simulink model "DWT"  (R2020a)
settings: Solver=ode45  StartTime=0.0  StopTime=4096+1024+100  RelTol=1e-3  EnableMultiTasking=on
PreLoadFcn:
  | xlrequire('imageData.mat'); xlrequire('PreLoadFcn');
PostLoadFcn:
  | open_system('DWT/Processor/Memory Controller','force'); pause(0.50); open_system('DWT');pause(0.50); close_system('DWT/Processor/Memory Controller');pause(0.50); close_system('DWT/Processor');
StopFcn:
  | xlrequire('StopFcn');
undefined symbols (not defined in the file or in its folder): b1Init, b2Init
libraries: xbsIndex_r4 x213, dspindex x4, dspsnks4 x2, dspmtrx3 x2, xbsCopyrightNotice_r4 x1, dspsrcs4 x1
(part 1 of 2)
settings Model: Creator=alexc  LastModifiedBy=viswanad
settings DataIOCC: LimitDataPoints=on  SaveFormat=Array  SignalLoggingSaveFormat=ModelDataLogs  ReturnWorkspaceOutputs=off  SignalLoggingName=sigsOut
settings OptimizationCC: BlockReduction=off  BooleanDataType=off  DefaultParameterBehavior=Inlined  ExpressionDepthLimit=2147483647  InitFltsAndDblsToZero=on  LifeSpan=inf
settings DebuggingCC: SaveWithParameterizedLinksMsg=none  UnderspecifiedInitializationDetection=Classic  MergeDetectMultiDrivingBlocksExec=none  SignalResolutionControl=TryResolveAllWithWarning  MultiTaskDSMMsg=warning  MultiTaskCondExecSysMsg=none  FcnCallInpInsideContextMsg=warning  AllowSymbolicDim=off  StateNameClashWarn=warning  SFUnexpectedBacktrackingDiag=warning  SFNoUnconditionalDefaultTransitionDiag=warning  SFExecutionAtInitializationDiag=none  ArithmeticOperatorsInVariantConditions=warning
settings HardwareCC: ProdBitPerPointer=32  ProdBitPerSizeT=32  ProdBitPerPtrDiffT=32  ProdLargestAtomicFloat=None  ProdIntDivRoundTo=Undefined  ProdEndianess=Unspecified  ProdWordSize=32  ProdHWDeviceType=32-bit Generic  TargetUnknown=on
settings ModelReferenceCC: PropagateSignalLabelsOutOfModel=off
settings SFSimCC: SimUseLocalCustomCode=off  CustomCodeUndefinedFunction=UseInterfaceOnly
settings RTWCC: Description=Generic Real-Time Target  RTWUseLocalCustomCode=off
settings CodeAppCC: StateflowObjectComments=on
settings GRTTargetCC: TargetFcnLib=ansi_tfl_tmw.mat  TargetLangStandard=C89/C90 (ANSI)  CombineOutputUpdateFcns=off  GRTInterface=on
settings ConfigComp: CovMetricSettings=dw  CovSaveCumulativeToWorkspaceVar=on  CovSaveSingleToWorkspaceVar=on  CovExternalEMLEnable=off

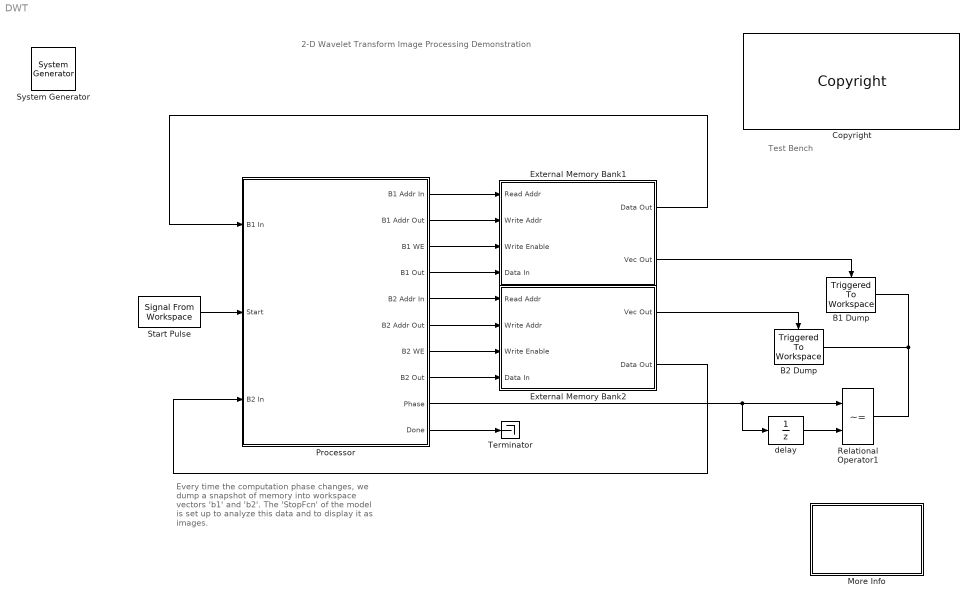
== system DWT ==
  note: Test
      |  Bench
  note: Every time the computation phase
      | changes, we dump a snapshot of
      | memory into workspace vectors  'b1'
      | and  'b2'.
      |
      | The 'StopFcn' of the model is set up
      | to analyze this data and to display
      | it as images.
  note: 2-D Wavelet Transform
      |  Image Processing Demonstration
  " System Generator" : xbsIndex_r4/ System Generator  Tag=genX  xilinxfamily=Kintex7  part=xc7k325t  speed=-3  package=fbg676  synthesis_tool=Vivado  clock_wrapper=Clock Enables  directory=./netlist  proj_type=Vivado  Synth_file=Vivado Synthesis Defaults  Impl_file=Vivado Implementation Defaults  testbench=off  simulink_period=1  sysclk_period=6  dcm_input_clock_period=10  incr_netlist=off  trim_vbits=Everywhere in SubSystem  dbl_ovrd=According to Block Masks  core_generation=According to Block Masks  run_coregen=off  deprecated_control=off  eval_field=0  block_type=sysgen
  B1 Dump : dspsnks4/Triggered To Workspace  TriggerType=Falling edge  VariableName=b1  Buffer=1000  Save2DMode=3-D array (concatenate along third dimension)
      settings: SourceProductBaseCode=DS  FixptAsFi=off
  B2 Dump : dspsnks4/Triggered To Workspace  TriggerType=Falling edge  VariableName=b2  Buffer=1000  Save2DMode=3-D array (concatenate along third dimension)
      settings: SourceProductBaseCode=DS  FixptAsFi=off
  Copyright : xbsCopyrightNotice_r4/Copyright  copyrighttext="Copyright (c) 2021  by  Xilinx, Inc. All rights reserved.<br><br>This file contains proprietary, confidential information of Xilinx, Inc., is distributed under license from Xilinx, Inc., and may be used, copied and/or disclosed only pursuant to the terms of a valid license agreement with Xilinx, Inc. Xilinx hereby grants you a license to use this file solely for design, simulation, implementation and creation of design files limited to Xilinx devices or technologies. Use with non-Xilinx devices or technologies is expressly prohibited and immediately terminates your license unless covered by a separate agreement.<br><br>Xilinx is providing this design, code, or information \"as-is\" solely for use in developing programs and solutions for Xilinx devices, with no obligation on the part of Xilinx to provide support. By providing this design, code, or information as one possible implementation of this feature, application or standard, Xilinx is making no representation that this implementation is free from any claims of infringement. You are responsible for obtaining any rights you may require for your implementation. Xilinx expressly disclaims any warranty whatsoever with respect to the adequacy of the implementation, including but not limited to any warranties or representations that this implementation is free from claims of infringement, implied warranties of merchantability or fitness for a particular purpose.<br><br>Xilinx products are not intended for use in life support appliances, devices, or systems. Use in such applications is expressly prohibited.<br><br>Any modifications that are made to the Source Code are done at the user's sole risk and will be unsupported.<br><br>This copyright and support notice must be retained as part of this text at all times. (c) Copyright 1995-2021 Xilinx, Inc. All rights reserved."  block_type=copyright
  External Memory Bank1 : Subsystem  mask{depth=size (b2Init, 2), init_vec=b1Init}
      mask prompts: depth "Memory Depth"; init_vec "Initial Value"
  External Memory Bank2 : Subsystem  mask{depth=size (b2Init, 2), init_vec=b2Init}
      mask prompts: depth "Memory Depth"; init_vec "Initial Value"
  More Info : Subsystem
      mask Display: disp('Double click\n for\n more information.')
  Processor : Subsystem
  Relational Operator1 : RelationalOperator  Operator=~=  RndMeth=Nearest  InputSameDT=on
  Start Pulse : dspsrcs4/Signal From Workspace  X=[ 0 0 0 1 0 0]  Ts=1  nsamps=1  OutputAfterFinalValue=Setting to zero  ignoreOrWarnInputAndFrameLengths=off  OutputFrames=on
  Terminator : Terminator
  delay : UnitDelay  InitialCondition=-1  HasFrameUpgradeWarning=on
  wires:
  Processor/4(B1 Out) -> External Memory Bank1/4(Data In)
  Processor/3(B1 WE) -> External Memory Bank1/3(Write Enable)
  Processor/2(B1 Addr Out) -> External Memory Bank1/2(Write Addr)
  Processor/1(B1 Addr In) -> External Memory Bank1/1(Read Addr)
  Processor/5(B2 Addr In) -> External Memory Bank2/1(Read Addr)
  Processor/6(B2 Addr Out) -> External Memory Bank2/2(Write Addr)
  Processor/7(B2 WE) -> External Memory Bank2/3(Write Enable)
  Processor/8(B2 Out) -> External Memory Bank2/4(Data In)
  External Memory Bank1/1(Data Out) -> Processor/1(B1 In)
  External Memory Bank2/2(Data Out) -> Processor/3(B2 In)
  External Memory Bank2/1(Vec Out) -> B2 Dump/1
  External Memory Bank1/2(Vec Out) -> B1 Dump/1
  Processor/9(Phase) -> Relational Operator1/1, delay/1
  delay/1 -> Relational Operator1/2
  Relational Operator1/1 -> B1 Dump/Trigger, B2 Dump/Trigger
  Start Pulse/1 -> Processor/2(Start)
  Processor/10(Done) -> Terminator/1

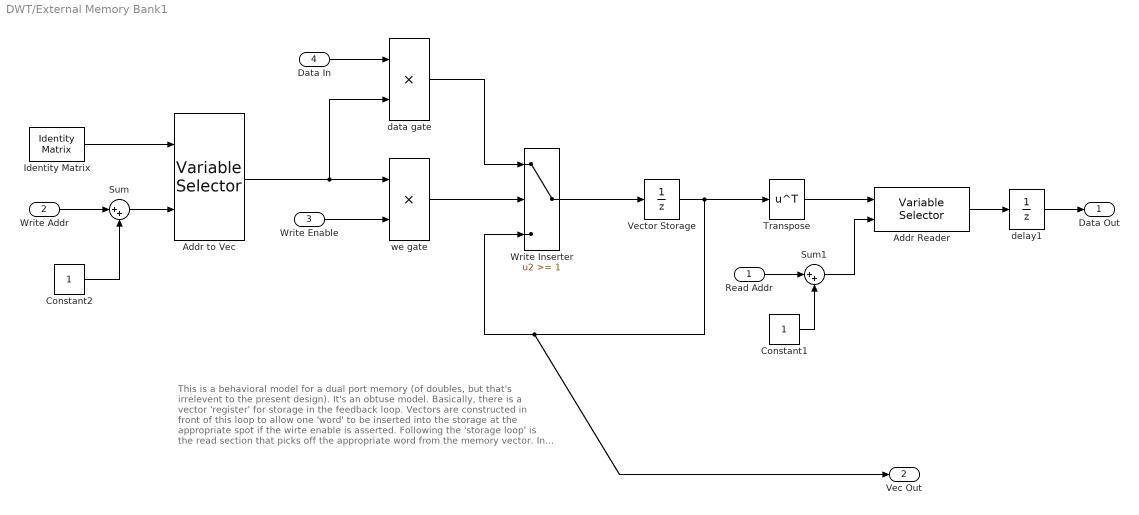
== system DWT/External Memory Bank1 ==
  note: This is a behavioral model for a dual port memory
      | (of doubles, but that's irrelevent to the present design).
      | It's an obtuse model.  Basically, there is a vector 'register'
      | for storage in the feedback loop. Vectors are constructed
      | in front of this loop to allow one 'word' to be inserted into the
      | storage  at the appropriate spot if the wirte enable is
      | asserted.  Following the 'storage loop' is the read section
      | that picks off the appropriate word from the memory vector.
      |
      | In case of overlapping addresss, the read is done before
      | the write changes the stored word.
      |
      | At every time step, the full contents of the memory are output
      | as a  vector of doubles.  This is a very handy  feature  for
      | analysis and debugging.
  Read Addr : Inport
  Write Addr : Inport  Port=2
  Write Enable : Inport  Port=3
  Data In : Inport  Port=4
  Addr Reader : dspindex/Variable Selector  NumInputs=1  rowsOrCols=Rows  IdxMode=Variable  Elements=[1 3]  ZerOneIdxMode=One-based  errmode=Generate Error  FillMode=on  FillValues=0
  Addr to Vec : dspindex/Variable Selector  NumInputs=1  rowsOrCols=Rows  IdxMode=Variable  Elements=[1 3]  ZerOneIdxMode=One-based  errmode=Clip Index  FillMode=on  FillValues=0
  Constant1 : Constant
  Constant2 : Constant
  Identity Matrix : dspmtrx3/Identity Matrix  Inherit=off  N=depth  Ts=1  dataType=double  isSigned=on  wordLen=16  udDataType=sfix(16)  fracBitsMode=Best precision  numFracBits=15  OutDataTypeStr=double  LastOutDataTypeStr=double
  Sum : Sum  Inputs=|++  InputSameDT=on  SaturateOnIntegerOverflow=on  OutDataTypeStr=Inherit: Same as first input
  Sum1 : Sum  Inputs=|++  InputSameDT=on  SaturateOnIntegerOverflow=on  OutDataTypeStr=Inherit: Same as first input
  Transpose : Math  Operator=transpose  SaturateOnIntegerOverflow=on
  Vector Storage : UnitDelay  InitialCondition=init_vec  HasFrameUpgradeWarning=on
  Write Inserter : Switch  Threshold=1  SaturateOnIntegerOverflow=on  InputSameDT=on
  data gate : Product  InputSameDT=on  SaturateOnIntegerOverflow=on  OutDataTypeStr=Inherit: Same as first input
  delay1 : UnitDelay  HasFrameUpgradeWarning=on
  we gate : Product  InputSameDT=on  SaturateOnIntegerOverflow=on  OutDataTypeStr=Inherit: Same as first input
  Data Out : Outport  VectorParamsAs1DForOutWhenUnconnected=off
  Vec Out : Outport  Port=2  VectorParamsAs1DForOutWhenUnconnected=off
  wires:
  Write Inserter/1 -> Vector Storage/1
  Addr Reader/1 -> delay1/1
  Addr to Vec/1 -> we gate/1, data gate/2
  Identity Matrix/1 -> Addr to Vec/1
  Write Enable/1 -> we gate/2
  Transpose/1 -> Addr Reader/1
  Data In/1 -> data gate/1
  we gate/1 -> Write Inserter/2
  data gate/1 -> Write Inserter/1
  Sum/1 -> Addr to Vec/2
  Write Addr/1 -> Sum/1
  Constant2/1 -> Sum/2
  Constant1/1 -> Sum1/2
  Sum1/1 -> Addr Reader/2
  delay1/1 -> Data Out/1
  Vector Storage/1 -> Transpose/1, Vec Out/1, Write Inserter/3
  Read Addr/1 -> Sum1/1

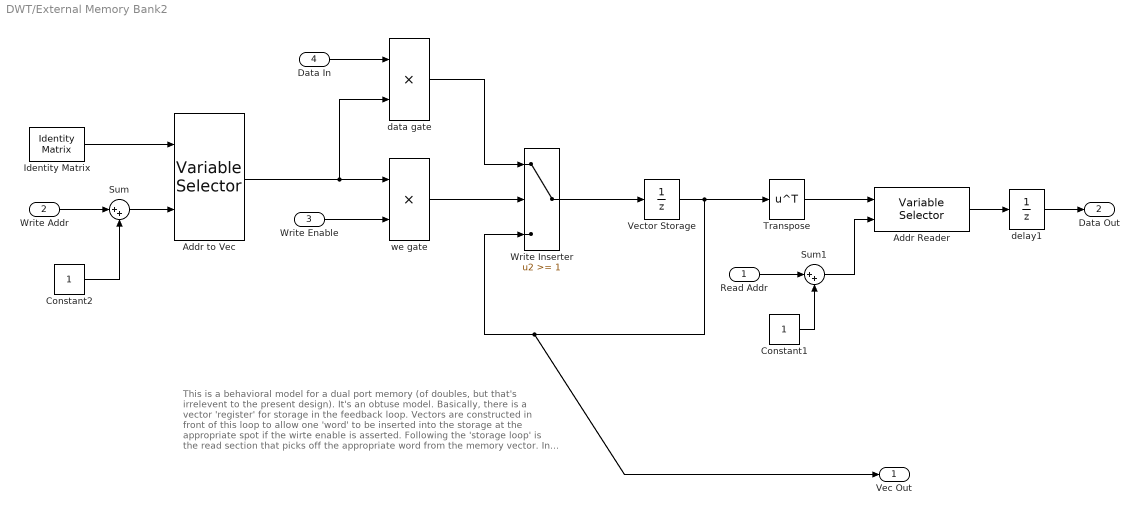
== system DWT/External Memory Bank2 ==
  note: This is a behavioral model for a dual port memory
      | (of doubles, but that's irrelevent to the present design).
      | It's an obtuse model.  Basically, there is a vector 'register'
      | for storage in the feedback loop. Vectors are constructed
      | in front of this loop to allow one 'word' to be inserted into the
      | storage  at the appropriate spot if the wirte enable is
      | asserted.  Following the 'storage loop' is the read section
      | that picks off the appropriate word from the memory vector.
      |
      | In case of overlapping addresss, the read is done before
      | the write changes the stored word.
      |
      | At every time step, the full contents of the memory are output
      | as a  vector of doubles.  This is a very handy  feature  for
      | analysis and debugging.
  Read Addr : Inport
  Write Addr : Inport  Port=2
  Write Enable : Inport  Port=3
  Data In : Inport  Port=4
  Addr Reader : dspindex/Variable Selector  NumInputs=1  rowsOrCols=Rows  IdxMode=Variable  Elements=[1 3]  ZerOneIdxMode=One-based  errmode=Clip Index  FillMode=on  FillValues=0
  Addr to Vec : dspindex/Variable Selector  NumInputs=1  rowsOrCols=Rows  IdxMode=Variable  Elements=[1 3]  ZerOneIdxMode=One-based  errmode=Clip Index  FillMode=on  FillValues=0
  Constant1 : Constant
  Constant2 : Constant
  Identity Matrix : dspmtrx3/Identity Matrix  Inherit=off  N=depth  Ts=1  dataType=double  isSigned=on  wordLen=16  udDataType=sfix(16)  fracBitsMode=Best precision  numFracBits=15  OutDataTypeStr=double  LastOutDataTypeStr=double
  Sum : Sum  Inputs=|++  InputSameDT=on  SaturateOnIntegerOverflow=on  OutDataTypeStr=Inherit: Same as first input
  Sum1 : Sum  Inputs=|++  InputSameDT=on  SaturateOnIntegerOverflow=on  OutDataTypeStr=Inherit: Same as first input
  Transpose : Math  Operator=transpose  SaturateOnIntegerOverflow=on
  Vector Storage : UnitDelay  InitialCondition=init_vec  HasFrameUpgradeWarning=on
  Write Inserter : Switch  Threshold=1  SaturateOnIntegerOverflow=on  InputSameDT=on
  data gate : Product  InputSameDT=on  SaturateOnIntegerOverflow=on  OutDataTypeStr=Inherit: Same as first input
  delay1 : UnitDelay  HasFrameUpgradeWarning=on
  we gate : Product  InputSameDT=on  SaturateOnIntegerOverflow=on  OutDataTypeStr=Inherit: Same as first input
  Vec Out : Outport  VectorParamsAs1DForOutWhenUnconnected=off
  Data Out : Outport  Port=2  VectorParamsAs1DForOutWhenUnconnected=off
  wires:
  Vector Storage/1 -> Transpose/1, Vec Out/1, Write Inserter/3
  delay1/1 -> Data Out/1
  Sum1/1 -> Addr Reader/2
  Read Addr/1 -> Sum1/1
  Constant1/1 -> Sum1/2
  Constant2/1 -> Sum/2
  Write Addr/1 -> Sum/1
  Sum/1 -> Addr to Vec/2
  data gate/1 -> Write Inserter/1
  we gate/1 -> Write Inserter/2
  Data In/1 -> data gate/1
  Transpose/1 -> Addr Reader/1
  Write Enable/1 -> we gate/2
  Identity Matrix/1 -> Addr to Vec/1
  Addr to Vec/1 -> data gate/2, we gate/1
  Addr Reader/1 -> delay1/1
  Write Inserter/1 -> Vector Storage/1

== system DWT/More Info ==
  note: The test bench for this wavelet design consists of a processor and behavioral models for a pair of external, dual-port memories.
      | The two memories are initialized with the pixel values of a grey-scale image.
      | The pixels from the initial image are interleaved into the two banks in a column first indexing strategy.
      | If the image contained a checkerboard of black and white pixels, then all of the black pixels will end up in the one bank, and all of
      | the white pixels in the other.  The processor includes a memory controller that schedules the reads and writes to memory, and
      | an image processing filter kernel that computes the 2D DWT decomposition of the image.  The processor has been configured
      | to compute two levels of decomposition on a 64 x 64 pixel image. The computation is done "in place" in the single image memory
      | space, and the initial pixel ordering is preserved throughout.
      |
      | A full color version of the design would easily fit in the same part as only the DWT datapath would require replication (the memoy
      | control could remain unchanged).
  note: 2-D Wavelet Transform Image Processing Demonstration

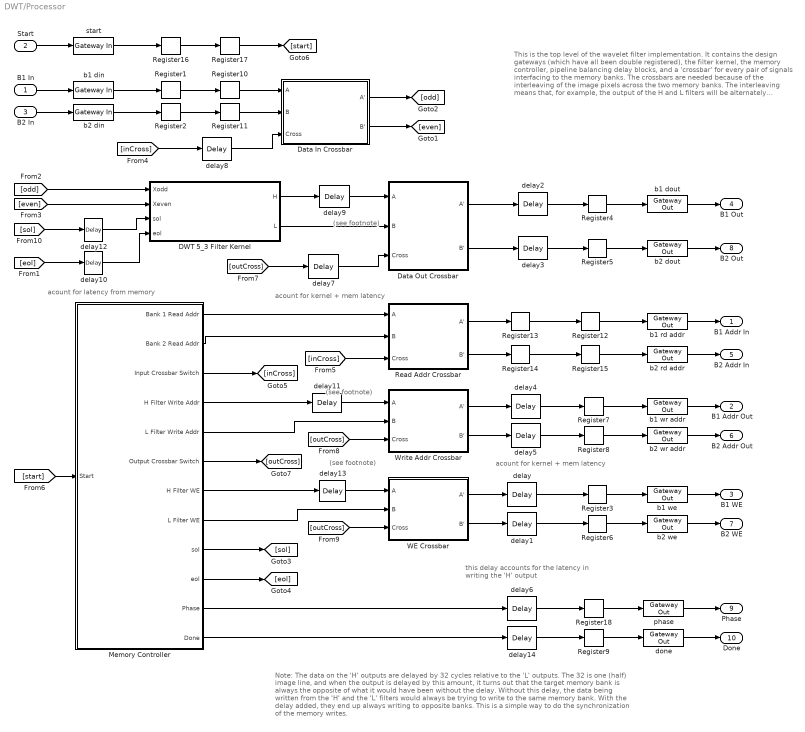
== system DWT/Processor ==
  note: This is the top level of the wavelet filter implementation.
      | It contains the design gateways (which have all been double
      | registered),  the filter kernel, the memory controller, pipeline
      | balancing delay blocks, and a 'crossbar' for every pair of signals
      | interfacing to the memory banks.  The crossbars are needed
      | because of the interleaving of the image pixels across the two
      | memory banks.  The interleaving means that, for example,
      | the output of the H and L filters will be alternately distributed
      | to the two memory banks.
  note: (see footnote)
  note: (see footnote)
  note: (see footnote)
  note: Note: The data on the 'H' outputs are delayed by 32 cycles relative to the 'L' outputs.
      | The 32 is one (half) image line, and when the output is delayed by this amount, it
      | turns out that the target memory bank is always the opposite of what it would have
      | been without the delay.  Without this delay, the data being written from the 'H' and
      | the 'L' filters would always be trying to write to the same memory bank.  With the
      | delay added, they end up always writing to opposite banks.  This is a simple way
      | to do the synchronization of the memory writes.
  note: this delay accounts for
      | the latency in writing the 'H' output
  note: acount for latency from memory
  note: acount for kernel + mem latency
  note: acount for kernel + mem latency
  B1 In : Inport
  Start : Inport  Port=2
  B2 In : Inport  Port=3
  DWT 5_3 Filter Kernel : Subsystem
  Data In Crossbar : Subsystem
  Data Out Crossbar : Subsystem
  Memory Controller : Subsystem  mask{N=6, M=6}
      mask prompts: N "Log Base 2 of Image Width"; M "Log Base 2 of Image Height"
  Read Addr Crossbar : Subsystem
  Register{1..18} (18 alike) : xbsIndex_r4/Register  init=0  rst=off  en=off  dbl_ovrd=off  block_type=register
  WE Crossbar : Subsystem
  Write Addr Crossbar : Subsystem
  b1 din : xbsIndex_r4/Gateway In  gui_display_data_type=Fixed-point  arith_type="Signed  (2's comp)"  n_bits=10  bin_pt=0  preci_type=Single  exp_width=8  frac_width=24  rows=1  columns=1  quantization="Round  (unbiased: +/- Inf)"  overflow=Saturate  period=1  UseAsADC=off  ADCChannel='1'  interface=None  automatic_assignment=on  address_offset=hex2dec('00')  intf_name=''  intf_description=''  default_value=0  timing_constraint=None  locs_specified=off  LOCs={}  io_standard={}  inherit_from_input=off  hdl_port=on  dbl_ovrd=off  block_type=gatewayin
  b1 dout : xbsIndex_r4/Gateway Out  inherit_from_input=off  hdl_port=on  rows=1  columns=1  UseAsDAC=off  DACChannel='1'  interface=None  automatic_assignment=on  address_offset=hex2dec('00')  intf_name=''  intf_description=''  timing_constraint=None  locs_specified=off  LOCs={}  io_standard={}  block_type=gatewayout
  b1 rd addr : xbsIndex_r4/Gateway Out  inherit_from_input=off  hdl_port=on  rows=1  columns=1  UseAsDAC=off  DACChannel='1'  interface=None  automatic_assignment=on  address_offset=hex2dec('00')  intf_name=''  intf_description=''  timing_constraint=None  locs_specified=off  LOCs={}  io_standard={}  block_type=gatewayout
  b1 we : xbsIndex_r4/Gateway Out  inherit_from_input=off  hdl_port=on  rows=1  columns=1  UseAsDAC=off  DACChannel='1'  interface=None  automatic_assignment=on  address_offset=hex2dec('00')  intf_name=''  intf_description=''  timing_constraint=None  locs_specified=off  LOCs={}  io_standard={}  block_type=gatewayout
  b1 wr addr : xbsIndex_r4/Gateway Out  inherit_from_input=off  hdl_port=on  rows=1  columns=1  UseAsDAC=off  DACChannel='1'  interface=None  automatic_assignment=on  address_offset=hex2dec('00')  intf_name=''  intf_description=''  timing_constraint=None  locs_specified=off  LOCs={}  io_standard={}  block_type=gatewayout
  b2 din : xbsIndex_r4/Gateway In  gui_display_data_type=Fixed-point  arith_type="Signed  (2's comp)"  n_bits=10  bin_pt=0  preci_type=Single  exp_width=8  frac_width=24  rows=1  columns=1  quantization="Round  (unbiased: +/- Inf)"  overflow=Saturate  period=1  UseAsADC=off  ADCChannel='1'  interface=None  automatic_assignment=on  address_offset=hex2dec('00')  intf_name=''  intf_description=''  default_value=0  timing_constraint=None  locs_specified=off  LOCs={}  io_standard={}  inherit_from_input=off  hdl_port=on  dbl_ovrd=off  block_type=gatewayin
  b2 dout : xbsIndex_r4/Gateway Out  inherit_from_input=off  hdl_port=on  rows=1  columns=1  UseAsDAC=off  DACChannel='1'  interface=None  automatic_assignment=on  address_offset=hex2dec('00')  intf_name=''  intf_description=''  timing_constraint=None  locs_specified=off  LOCs={}  io_standard={}  block_type=gatewayout
  b2 rd addr : xbsIndex_r4/Gateway Out  inherit_from_input=off  hdl_port=on  rows=1  columns=1  UseAsDAC=off  DACChannel='1'  interface=None  automatic_assignment=on  address_offset=hex2dec('00')  intf_name=''  intf_description=''  timing_constraint=None  locs_specified=off  LOCs={}  io_standard={}  block_type=gatewayout
  b2 we : xbsIndex_r4/Gateway Out  inherit_from_input=off  hdl_port=on  rows=1  columns=1  UseAsDAC=off  DACChannel='1'  interface=None  automatic_assignment=on  address_offset=hex2dec('00')  intf_name=''  intf_description=''  timing_constraint=None  locs_specified=off  LOCs={}  io_standard={}  block_type=gatewayout
  b2 wr addr : xbsIndex_r4/Gateway Out  inherit_from_input=off  hdl_port=on  rows=1  columns=1  UseAsDAC=off  DACChannel='1'  interface=None  automatic_assignment=on  address_offset=hex2dec('00')  intf_name=''  intf_description=''  timing_constraint=None  locs_specified=off  LOCs={}  io_standard={}  block_type=gatewayout
  delay{,1,4..5} (4 alike) : xbsIndex_r4/Delay  rst=off  infoeditControl=Selection of Reset will increase slice count due to use of real FFs and instead of SRLs  en=off  latency=15  reg_retiming=off  dbl_ovrd=off  block_type=delay
  delay10 : xbsIndex_r4/Delay  rst=off  infoeditControl=Selection of Reset will increase slice count due to use of real FFs and instead of SRLs  en=off  latency=6  reg_retiming=off  dbl_ovrd=off  block_type=delay
  delay11 : xbsIndex_r4/Delay  rst=off  infoeditControl=Selection of Reset will increase slice count due to use of real FFs and instead of SRLs  en=off  latency=32  reg_retiming=off  dbl_ovrd=off  block_type=delay
  delay12 : xbsIndex_r4/Delay  rst=off  infoeditControl=Selection of Reset will increase slice count due to use of real FFs and instead of SRLs  en=off  latency=6  reg_retiming=off  dbl_ovrd=off  block_type=delay
  delay13 : xbsIndex_r4/Delay  rst=off  infoeditControl=Selection of Reset will increase slice count due to use of real FFs and instead of SRLs  en=off  latency=32  reg_retiming=off  dbl_ovrd=off  block_type=delay
  delay14 : xbsIndex_r4/Delay  rst=off  infoeditControl=Selection of Reset will increase slice count due to use of real FFs and instead of SRLs  en=off  latency=32+15  reg_retiming=off  dbl_ovrd=off  block_type=delay
  delay2 : xbsIndex_r4/Delay  rst=off  infoeditControl=Selection of Reset will increase slice count due to use of real FFs and instead of SRLs  en=off  latency=1  reg_retiming=off  dbl_ovrd=off  block_type=delay
  delay3 : xbsIndex_r4/Delay  rst=off  infoeditControl=Selection of Reset will increase slice count due to use of real FFs and instead of SRLs  en=off  latency=1  reg_retiming=off  dbl_ovrd=off  block_type=delay
  delay6 : xbsIndex_r4/Delay  rst=off  infoeditControl=Selection of Reset will increase slice count due to use of real FFs and instead of SRLs  en=off  latency=32+15  reg_retiming=off  dbl_ovrd=off  block_type=delay
  delay7 : xbsIndex_r4/Delay  rst=off  infoeditControl=Selection of Reset will increase slice count due to use of real FFs and instead of SRLs  en=off  latency=14  reg_retiming=off  dbl_ovrd=off  block_type=delay
  delay8 : xbsIndex_r4/Delay  rst=off  infoeditControl=Selection of Reset will increase slice count due to use of real FFs and instead of SRLs  en=off  latency=6  reg_retiming=off  dbl_ovrd=off  block_type=delay
  delay9 : xbsIndex_r4/Delay  rst=off  infoeditControl=Selection of Reset will increase slice count due to use of real FFs and instead of SRLs  en=off  latency=32  reg_retiming=off  dbl_ovrd=off  block_type=delay
  done : xbsIndex_r4/Gateway Out  inherit_from_input=off  hdl_port=on  rows=1  columns=1  UseAsDAC=off  DACChannel='1'  interface=None  automatic_assignment=on  address_offset=hex2dec('00')  intf_name=''  intf_description=''  timing_constraint=None  locs_specified=off  LOCs={}  io_standard={}  block_type=gatewayout
  phase : xbsIndex_r4/Gateway Out  inherit_from_input=off  hdl_port=on  rows=1  columns=1  UseAsDAC=off  DACChannel='1'  interface=None  automatic_assignment=on  address_offset=hex2dec('00')  intf_name=''  intf_description=''  timing_constraint=None  locs_specified=off  LOCs={}  io_standard={}  block_type=gatewayout
  start : xbsIndex_r4/Gateway In  gui_display_data_type=Boolean  arith_type=Boolean  n_bits=1  bin_pt=0  preci_type=Single  exp_width=8  frac_width=24  rows=1  columns=1  quantization="Round  (unbiased: +/- Inf)"  overflow=Saturate  period=1  UseAsADC=off  ADCChannel='1'  interface=None  automatic_assignment=on  address_offset=hex2dec('00')  intf_name=''  intf_description=''  default_value=0  timing_constraint=None  locs_specified=off  LOCs={}  io_standard={}  inherit_from_input=off  hdl_port=on  dbl_ovrd=off  block_type=gatewayin
  B1 Addr In : Outport  VectorParamsAs1DForOutWhenUnconnected=off
  B1 Addr Out : Outport  Port=2  VectorParamsAs1DForOutWhenUnconnected=off
  B1 WE : Outport  Port=3  VectorParamsAs1DForOutWhenUnconnected=off
  B1 Out : Outport  Port=4  VectorParamsAs1DForOutWhenUnconnected=off
  B2 Addr In : Outport  Port=5  VectorParamsAs1DForOutWhenUnconnected=off
  B2 Addr Out : Outport  Port=6  VectorParamsAs1DForOutWhenUnconnected=off
  B2 WE : Outport  Port=7  VectorParamsAs1DForOutWhenUnconnected=off
  B2 Out : Outport  Port=8  VectorParamsAs1DForOutWhenUnconnected=off
  Phase : Outport  Port=9  VectorParamsAs1DForOutWhenUnconnected=off
  Done : Outport  Port=10  VectorParamsAs1DForOutWhenUnconnected=off
  wires:
  b1 din/1 -> Register1/1
  b2 din/1 -> Register2/1
  [sol] -> delay12/1
  [eol] -> delay10/1
  [odd] -> DWT 5_3 Filter Kernel/1(Xodd)
  [even] -> DWT 5_3 Filter Kernel/2(Xeven)
  Register1/1 -> Register10/1
  Register2/1 -> Register11/1
  Memory Controller/5(L Filter Write Addr) -> Write Addr Crossbar/2(B)
  Memory Controller/4(H Filter Write Addr) -> delay11/1
  Memory Controller/11(Phase) -> delay6/1
  Memory Controller/9(sol) -> [sol]
  Memory Controller/10(eol) -> [eol]
  Write Addr Crossbar/1(A') -> delay4/1
  Write Addr Crossbar/2(B') -> delay5/1
  DWT 5_3 Filter Kernel/1(H) -> delay9/1
  DWT 5_3 Filter Kernel/2(L) -> Data Out Crossbar/2(B)
  Data Out Crossbar/1(A') -> delay2/1
  Data Out Crossbar/2(B') -> delay3/1
  Register4/1 -> b1 dout/1
  Register5/1 -> b2 dout/1
  b2 rd addr/1 -> B2 Addr In/1
  b1 wr addr/1 -> B1 Addr Out/1
  b2 wr addr/1 -> B2 Addr Out/1
  B1 In/1 -> b1 din/1
  B2 In/1 -> b2 din/1
  b1 dout/1 -> B1 Out/1
  b2 dout/1 -> B2 Out/1
  b1 we/1 -> B1 WE/1
  b2 we/1 -> B2 WE/1
  delay2/1 -> Register4/1
  delay3/1 -> Register5/1
  delay5/1 -> Register8/1
  delay4/1 -> Register7/1
  Register7/1 -> b1 wr addr/1
  Register8/1 -> b2 wr addr/1
  phase/1 -> Phase/1
  Data In Crossbar/1(A') -> [odd]
  Data In Crossbar/2(B') -> [even]
  Memory Controller/3(Input Crossbar Switch) -> [inCross]
  Read Addr Crossbar/1(A') -> Register13/1
  Read Addr Crossbar/2(B') -> Register14/1
  Memory Controller/2(Bank 2 Read Addr) -> Read Addr Crossbar/2(B)
  Memory Controller/1(Bank 1 Read Addr) -> Read Addr Crossbar/1(A)
  delay6/1 -> Register18/1
  delay7/1 -> Data Out Crossbar/3(Cross)
  delay8/1 -> Data In Crossbar/3(Cross)
  [inCross] -> delay8/1
  [inCross] -> Read Addr Crossbar/3(Cross)
  delay10/1 -> DWT 5_3 Filter Kernel/4(eol)
  delay12/1 -> DWT 5_3 Filter Kernel/3(sol)
  delay9/1 -> Data Out Crossbar/1(A)
  delay11/1 -> Write Addr Crossbar/1(A)
  delay1/1 -> Register6/1
  delay/1 -> Register3/1
  WE Crossbar/2(B') -> delay1/1
  WE Crossbar/1(A') -> delay/1
  delay13/1 -> WE Crossbar/1(A)
  Register3/1 -> b1 we/1
  Register6/1 -> b2 we/1
  Register10/1 -> Data In Crossbar/1(A)
  Register11/1 -> Data In Crossbar/2(B)
  Register12/1 -> b1 rd addr/1
  Register13/1 -> Register12/1
  Register14/1 -> Register15/1
  Register15/1 -> b2 rd addr/1
  Start/1 -> start/1
  start/1 -> Register16/1
  Register16/1 -> Register17/1
  Register17/1 -> [start]
  [start] -> Memory Controller/1(Start)
  Memory Controller/6(Output Crossbar Switch) -> [outCross]
  [outCross] -> delay7/1
  [outCross] -> Write Addr Crossbar/3(Cross)
  [outCross] -> WE Crossbar/3(Cross)
  done/1 -> Done/1
  delay14/1 -> Register9/1
  Register9/1 -> done/1
  Register18/1 -> phase/1
  Memory Controller/12(Done) -> delay14/1
  b1 rd addr/1 -> B1 Addr In/1
  Memory Controller/7(H Filter WE) -> delay13/1
  Memory Controller/8(L Filter WE) -> WE Crossbar/2(B)

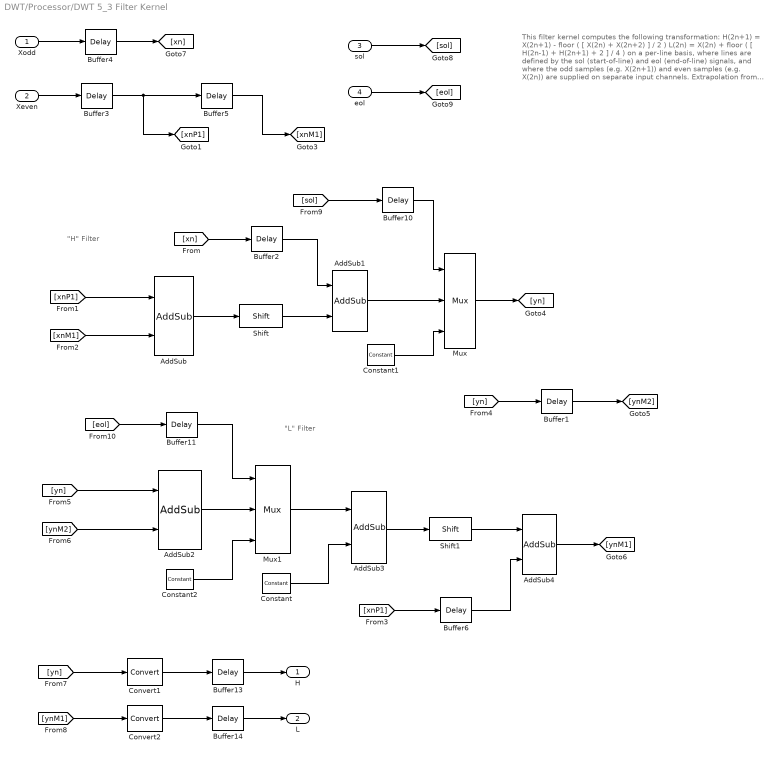
== system DWT/Processor/DWT 5_3 Filter Kernel ==
  note: This filter kernel computes the following transformation:
      |
      |    H(2n+1) = X(2n+1) - floor ( [ X(2n) + X(2n+2) ] / 2 )
      |    L(2n)      =  X(2n)  + floor ( [ H(2n-1) + H(2n+1) + 2 ] / 4 )
      |
      | on a per-line basis, where lines are defined by the sol
      | (start-of-line) and eol (end-of-line) signals, and where
      | the odd samples (e.g. X(2n+1)) and even samples
      | (e.g. X(2n)) are supplied on separate input channels.
      |
      | Extrapolation from the endpoints of the line is required
      | to compute the above transformation.  We have chosen
      | a Neuman extrapolation, wherein, effectively, the second
      | derivative of the data becomes zero at the endpoint and
      | the data is inflected.  Thus, with x(1) being an endpoint,
      | we construct:
      |    X(0) = X(1) - [ X(2) - X(1) ]        and
      |    X(-1) = X(1) - 2 [ X(3) - X(1) ]
      |
      | This extrapolation scheme becomes very simple in
      | the hardware implementation, adding only the two muxes
      | appearing below.
  note: "H" Filter
  note: "L" Filter
  Xodd : Inport
  Xeven : Inport  Port=2
  sol : Inport  Port=3
  eol : Inport  Port=4
  AddSub{,2..4} (4 alike) : xbsIndex_r4/AddSub  mode=Addition  use_carryin=off  use_carryout=off  en=off  latency=1  precision=Full  arith_type=Unsigned  n_bits=8  bin_pt=2  quantization=Truncate  overflow=Wrap  use_behavioral_HDL=on  hw_selection=Fabric  pipelined=off  use_rpm=off  XmcBlockStatus=1  maskContainerNames=tabcontainer1  block_type=addsub  block_config=sysgen:Addsub_config
  AddSub1 : xbsIndex_r4/AddSub  mode=Subtraction  use_carryin=off  use_carryout=off  en=off  latency=1  precision=Full  arith_type=Unsigned  n_bits=8  bin_pt=2  quantization=Truncate  overflow=Wrap  use_behavioral_HDL=on  hw_selection=Fabric  pipelined=off  use_rpm=off  XmcBlockStatus=1  maskContainerNames=tabcontainer1  block_type=addsub  block_config=sysgen:Addsub_config
  Buffer{1..5,14} (6 alike) : xbsIndex_r4/Delay  rst=off  en=off  latency=1  reg_retiming=off  XmcBlockStatus=1  maskContainerNames=group1  block_type=delay  block_config=sysgen:Delay_config
  Buffer10 : xbsIndex_r4/Delay  rst=off  en=off  latency=3  reg_retiming=off  XmcBlockStatus=1  maskContainerNames=group1  block_type=delay  block_config=sysgen:Delay_config
  Buffer11 : xbsIndex_r4/Delay  rst=off  en=off  latency=7  reg_retiming=off  XmcBlockStatus=1  maskContainerNames=group1  block_type=delay  block_config=sysgen:Delay_config
  Buffer13 : xbsIndex_r4/Delay  rst=off  en=off  latency=6  reg_retiming=off  XmcBlockStatus=1  maskContainerNames=group1  block_type=delay  block_config=sysgen:Delay_config
  Buffer6 : xbsIndex_r4/Delay  rst=off  en=off  latency=5  reg_retiming=off  XmcBlockStatus=1  maskContainerNames=group1  block_type=delay  block_config=sysgen:Delay_config
  Constant : xbsIndex_r4/Constant  const=2  gui_display_data_type=Fixed-point  arith_type=Unsigned  n_bits=2  bin_pt=0  preci_type=Single  exp_width=8  frac_width=24  explicit_period=off  period=1  XmcBlockStatus=1  maskContainerNames=tabcontainer1  block_type=constant  block_config=sysgen:Constant_config
  Constant1 : xbsIndex_r4/Constant  const=0  gui_display_data_type=Fixed-point  arith_type=Signed (2's comp)  n_bits=11  bin_pt=0  preci_type=Single  exp_width=8  frac_width=24  explicit_period=off  period=1  XmcBlockStatus=1  maskContainerNames=tabcontainer1  block_type=constant  block_config=sysgen:Constant_config
  Constant2 : xbsIndex_r4/Constant  const=0  gui_display_data_type=Fixed-point  arith_type=Signed (2's comp)  n_bits=12  bin_pt=0  preci_type=Single  exp_width=8  frac_width=24  explicit_period=off  period=1  XmcBlockStatus=1  maskContainerNames=tabcontainer1  block_type=constant  block_config=sysgen:Constant_config
  Convert1 : xbsIndex_r4/Convert  gui_display_data_type=Fixed-point  arith_type="Signed  (2's comp)"  n_bits=10  bin_pt=0  float_type=Single  exp_bits=8  fraction_bits=24  quantization="Round  (unbiased: +/- Inf)"  overflow=Saturate  en=off  latency=0  pipeline=off  XmcBlockStatus=1  maskContainerNames=group2  block_type=convert  block_config=sysgen:Convert_config
  Convert2 : xbsIndex_r4/Convert  gui_display_data_type=Fixed-point  arith_type="Signed  (2's comp)"  n_bits=10  bin_pt=0  float_type=Single  exp_bits=8  fraction_bits=24  quantization="Round  (unbiased: +/- Inf)"  overflow=Saturate  en=off  latency=0  pipeline=off  XmcBlockStatus=1  maskContainerNames=group2  block_type=convert  block_config=sysgen:Convert_config
  Mux : xbsIndex_r4/Mux  inputs=2  en=off  latency=1  precision=Full  arith_type="Signed  (2's comp)"  n_bits=8  bin_pt=2  quantization=Truncate  overflow=Wrap  XmcBlockStatus=1  maskContainerNames=tabcontainer1  block_type=mux  block_config=sysgen:Mux_config
      settings: infoedit=[]
  Mux1 : xbsIndex_r4/Mux  inputs=2  en=off  latency=1  precision=Full  arith_type="Signed  (2's comp)"  n_bits=8  bin_pt=2  quantization=Truncate  overflow=Wrap  XmcBlockStatus=1  maskContainerNames=tabcontainer1  block_type=mux  block_config=sysgen:Mux_config
      settings: infoedit=[]
  Shift : xbsIndex_r4/Shift  shift_dir=Right  shift_bits=1  en=off  latency=0  precision=User Defined  arith_type="Signed  (2's comp)"  n_bits=10  bin_pt=0  quantization=Truncate  overflow=Wrap  XmcBlockStatus=1  maskContainerNames=group2  block_type=shift  block_config=sysgen:Shift_config
  Shift1 : xbsIndex_r4/Shift  shift_dir=Right  shift_bits=2  en=off  latency=0  precision=User Defined  arith_type="Signed  (2's comp)"  n_bits=11  bin_pt=0  quantization=Truncate  overflow=Wrap  XmcBlockStatus=1  maskContainerNames=group2  block_type=shift  block_config=sysgen:Shift_config
  H : Outport  VectorParamsAs1DForOutWhenUnconnected=off
  L : Outport  Port=2  VectorParamsAs1DForOutWhenUnconnected=off
  wires:
  Buffer6/1 -> AddSub4/2
  Buffer2/1 -> AddSub1/1
  Buffer11/1 -> Mux1/1
  Constant2/1 -> Mux1/3
  AddSub2/1 -> Mux1/2
  Mux1/1 -> AddSub3/1
  AddSub4/1 -> [ynM1]
  Buffer14/1 -> L/1
  Buffer13/1 -> H/1
  [xnP1] -> Buffer6/1
  Shift1/1 -> AddSub4/1
  [eol] -> Buffer11/1
  AddSub3/1 -> Shift1/1
  Buffer10/1 -> Mux/1
  [sol] -> Buffer10/1
  Constant1/1 -> Mux/3
  AddSub1/1 -> Mux/2
  Mux/1 -> [yn]
  sol/1 -> [sol]
  Xodd/1 -> Buffer4/1
  Xeven/1 -> Buffer3/1
  [xn] -> Buffer2/1
  Convert2/1 -> Buffer14/1
  Convert1/1 -> Buffer13/1
  [ynM1] -> Convert2/1
  [yn] -> Convert1/1
  [ynM2] -> AddSub2/2
  [yn] -> AddSub2/1
  Buffer1/1 -> [ynM2]
  [yn] -> Buffer1/1
  Buffer5/1 -> [xnM1]
  Buffer3/1 -> [xnP1], Buffer5/1
  [xnP1] -> AddSub/1
  [xnM1] -> AddSub/2
  AddSub/1 -> Shift/1
  Shift/1 -> AddSub1/2
  Constant/1 -> AddSub3/2
  eol/1 -> [eol]
  Buffer4/1 -> [xn]

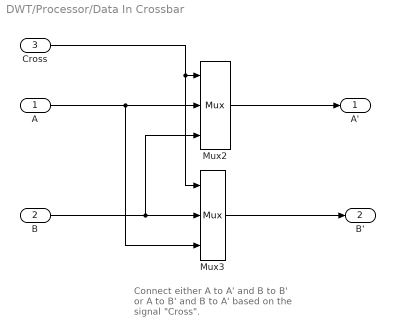
== system DWT/Processor/Data In Crossbar ==
  note: Connect either A to A' and B to B'
      | or A to B' and B to A' based on
      | the signal "Cross".
  A : Inport
  B : Inport  Port=2
  Cross : Inport  Port=3
  Mux2 : xbsIndex_r4/Mux  inputs=2  en=off  latency=1  precision=Full  arith_type="Signed  (2's comp)"  n_bits=8  bin_pt=2  quantization=Truncate  overflow=Wrap  XmcBlockStatus=1  maskContainerNames=tabcontainer1  block_type=mux  block_config=sysgen:Mux_config
      settings: infoedit=[]
  Mux3 : xbsIndex_r4/Mux  inputs=2  en=off  latency=1  precision=Full  arith_type="Signed  (2's comp)"  n_bits=8  bin_pt=2  quantization=Truncate  overflow=Wrap  XmcBlockStatus=1  maskContainerNames=tabcontainer1  block_type=mux  block_config=sysgen:Mux_config
      settings: infoedit=[]
  A' : Outport  VectorParamsAs1DForOutWhenUnconnected=off
  B' : Outport  Port=2  VectorParamsAs1DForOutWhenUnconnected=off
  wires:
  Mux2/1 -> A'/1
  Mux3/1 -> B'/1
  A/1 -> Mux2/2, Mux3/3
  B/1 -> Mux3/2, Mux2/3
  Cross/1 -> Mux2/1, Mux3/1

== system DWT/Processor/Data Out Crossbar ==
  note: Connect either A to A' and B to B'
      | or A to B' and B to A' based on
      | the signal "Cross".
  A : Inport
  B : Inport  Port=2
  Cross : Inport  Port=3
  Mux2 : xbsIndex_r4/Mux  inputs=2  en=off  latency=1  precision=Full  arith_type="Signed  (2's comp)"  n_bits=8  bin_pt=2  quantization=Truncate  overflow=Wrap  XmcBlockStatus=1  maskContainerNames=tabcontainer1  block_type=mux  block_config=sysgen:Mux_config
      settings: infoedit=[]
  Mux3 : xbsIndex_r4/Mux  inputs=2  en=off  latency=1  precision=Full  arith_type="Signed  (2's comp)"  n_bits=8  bin_pt=2  quantization=Truncate  overflow=Wrap  XmcBlockStatus=1  maskContainerNames=tabcontainer1  block_type=mux  block_config=sysgen:Mux_config
      settings: infoedit=[]
  A' : Outport  VectorParamsAs1DForOutWhenUnconnected=off
  B' : Outport  Port=2  VectorParamsAs1DForOutWhenUnconnected=off
  wires:
  Cross/1 -> Mux3/1, Mux2/1
  B/1 -> Mux2/3, Mux3/2
  A/1 -> Mux3/3, Mux2/2
  Mux3/1 -> B'/1
  Mux2/1 -> A'/1

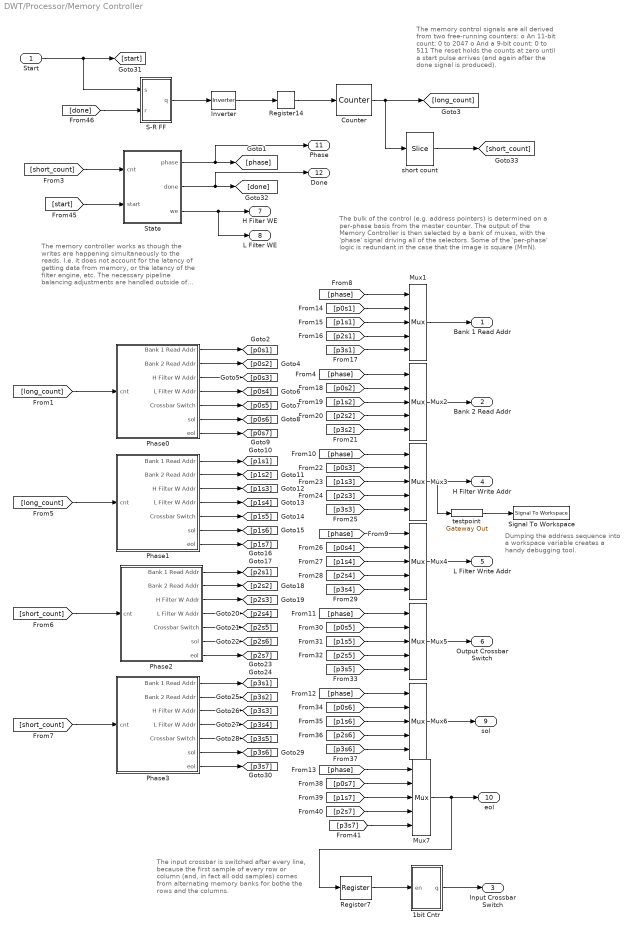
== system DWT/Processor/Memory Controller ==
  note: The memory control signals are all
      | derived from two free-running counters:
      |   o  An 11-bit count:    0 to 2047
      |   o  And a 9-bit count: 0 to 511
      | The reset holds the counts at zero until
      | a start pulse arrives (and again after the
      | done signal is produced).
  note: The bulk of the control (e.g. address pointers) is determined
      | on a per-phase basis from the master counter.  The output of
      | the Memory Controller is then selected by a bank of muxes,
      | with the 'phase' signal driving all of the selectors.  Some of
      | the 'per-phase' logic is redundant in the case that the image
      | is square (M=N).
  note: The memory controller works as though the
      | writes are happening simultaneously to the
      | reads. I.e. it does not account for the latency
      | of getting data from memory, or the latency
      | of the filter engine, etc.  The necessary
      | pipeline balancing adjustments are handled
      | outside of the controller.  This makes for a
      | much simpler control structure.
  note: The input crossbar is switched after every
      | line, because the first sample of every
      | row or column (and, in fact all odd samples)
      | comes from alternating memory banks for
      | bothe the rows and the columns.
  note: Dumping the address sequence
      | into a workspace variable creates
      | a handy debugging tool.
  Start : Inport
  1bit Cntr : Subsystem
  Counter : xbsIndex_r4/Counter  cnt_type=Free Running  cnt_to=Inf  operation=Up  start_count=0  cnt_by_val=1  arith_type=Unsigned  n_bits=N+M-1  bin_pt=0  load_pin=off  rst=on  en=off  explicit_period=off  period=1  use_behavioral_HDL=off  implementation=Fabric  use_rpm=off  dbl_ovrd=off  block_type=counter
  Inverter : xbsIndex_r4/Inverter  en=off  latency=0  dbl_ovrd=off  block_type=inv
  Mux{1..7} (7 alike) : xbsIndex_r4/Mux  inputs=4  en=off  latency=1  precision=Full  arith_type="Signed  (2's comp)"  n_bits=8  bin_pt=2  quantization=Truncate  overflow=Wrap  dbl_ovrd=off  block_type=mux
      settings: infoedit=[]
  Phase0 : Subsystem
  Phase1 : Subsystem
  Phase2 : Subsystem
  Phase3 : Subsystem
  Register14 : xbsIndex_r4/Register  init=1  rst=off  en=off  dbl_ovrd=off  block_type=register
  Register7 : xbsIndex_r4/Register  init=0  rst=off  en=off  dbl_ovrd=off  block_type=register
  S-R FF : Subsystem
  Signal To Workspace : SignalToWorkspace  VariableName=HWriteAddr
      settings: CopyFcn=dspblkcopystw(gcbh);  Save2DSignal=3-D array (concatenate along third dimension)
  State : Subsystem
  short count : xbsIndex_r4/Slice  nbits=M+N-3  boolean_output=off  mode=Lower Bit Location + Width  bit1=0  base1=MSB of Input  bit0=0  base0=LSB of Input  dbl_ovrd=off  block_type=slice
  testpoint : xbsIndex_r4/Gateway Out  inherit_from_input=off  hdl_port=off  rows=1  columns=1  UseAsDAC=off  DACChannel='1'  interface=None  automatic_assignment=on  address_offset=hex2dec('00')  intf_name=''  intf_description=''  timing_constraint=None  locs_specified=off  LOCs={}  io_standard={}  block_type=gatewayout
  Bank 1 Read Addr : Outport  VectorParamsAs1DForOutWhenUnconnected=off
  Bank 2 Read Addr : Outport  Port=2  VectorParamsAs1DForOutWhenUnconnected=off
  Input Crossbar Switch : Outport  Port=3  VectorParamsAs1DForOutWhenUnconnected=off
  H Filter Write Addr : Outport  Port=4  VectorParamsAs1DForOutWhenUnconnected=off
  L Filter Write Addr : Outport  Port=5  VectorParamsAs1DForOutWhenUnconnected=off
  Output Crossbar Switch : Outport  Port=6  VectorParamsAs1DForOutWhenUnconnected=off
  H Filter WE : Outport  Port=7  VectorParamsAs1DForOutWhenUnconnected=off
  L Filter WE : Outport  Port=8  VectorParamsAs1DForOutWhenUnconnected=off
  sol : Outport  Port=9  VectorParamsAs1DForOutWhenUnconnected=off
  eol : Outport  Port=10  VectorParamsAs1DForOutWhenUnconnected=off
  Phase : Outport  Port=11  VectorParamsAs1DForOutWhenUnconnected=off
  Done : Outport  Port=12  VectorParamsAs1DForOutWhenUnconnected=off
  wires:
  Counter/1 -> [long_count], short count/1
  [long_count] -> Phase0/1(cnt)
  State/1(phase) -> Phase/1, [phase]
  [long_count] -> Phase1/1(cnt)
  [short_count] -> Phase2/1(cnt)
  [short_count] -> Phase3/1(cnt)
  [phase] -> Mux1/1
  [phase] -> Mux2/1
  [phase] -> Mux3/1
  [phase] -> Mux4/1
  [phase] -> Mux5/1
  [phase] -> Mux6/1
  [phase] -> Mux7/1
  Phase0/1(Bank 1 Read Addr) -> [p0s1]
  Phase0/2(Bank 2 Read Addr) -> [p0s2]
  Phase0/3(H Filter W Addr) -> [p0s3]
  Phase0/4(L Filter W Addr) -> [p0s4]
  Phase0/5(Crossbar Switch) -> [p0s5]
  Phase0/6(sol) -> [p0s6]
  Phase0/7(eol) -> [p0s7]
  Phase1/1(Bank 1 Read Addr) -> [p1s1]
  Phase1/2(Bank 2 Read Addr) -> [p1s2]
  Phase1/3(H Filter W Addr) -> [p1s3]
  Phase1/4(L Filter W Addr) -> [p1s4]
  Phase1/5(Crossbar Switch) -> [p1s5]
  Phase1/6(sol) -> [p1s6]
  Phase1/7(eol) -> [p1s7]
  Phase2/1(Bank 1 Read Addr) -> [p2s1]
  Phase2/2(Bank 2 Read Addr) -> [p2s2]
  Phase2/3(H Filter W Addr) -> [p2s3]
  Phase2/4(L Filter W Addr) -> [p2s4]
  Phase2/5(Crossbar Switch) -> [p2s5]
  Phase2/6(sol) -> [p2s6]
  Phase2/7(eol) -> [p2s7]
  Phase3/1(Bank 1 Read Addr) -> [p3s1]
  Phase3/2(Bank 2 Read Addr) -> [p3s2]
  Phase3/3(H Filter W Addr) -> [p3s3]
  Phase3/4(L Filter W Addr) -> [p3s4]
  Phase3/5(Crossbar Switch) -> [p3s5]
  Phase3/6(sol) -> [p3s6]
  Phase3/7(eol) -> [p3s7]
  [p0s1] -> Mux1/2
  [p1s1] -> Mux1/3
  [p2s1] -> Mux1/4
  [p3s1] -> Mux1/5
  [p0s2] -> Mux2/2
  [p1s2] -> Mux2/3
  [p2s2] -> Mux2/4
  [p3s2] -> Mux2/5
  [p0s3] -> Mux3/2
  [p1s3] -> Mux3/3
  [p2s3] -> Mux3/4
  [p3s3] -> Mux3/5
  [p0s4] -> Mux4/2
  [p1s4] -> Mux4/3
  [p2s4] -> Mux4/4
  [p3s4] -> Mux4/5
  [p0s5] -> Mux5/2
  [p1s5] -> Mux5/3
  [p2s5] -> Mux5/4
  [p3s5] -> Mux5/5
  [p0s6] -> Mux6/2
  [p1s6] -> Mux6/3
  [p2s6] -> Mux6/4
  [p3s6] -> Mux6/5
  [p0s7] -> Mux7/2
  [p1s7] -> Mux7/3
  [p2s7] -> Mux7/4
  [p3s7] -> Mux7/5
  Mux7/1 -> eol/1, Register7/1
  Mux6/1 -> sol/1
  Mux5/1 -> Output Crossbar Switch/1
  Mux4/1 -> L Filter Write Addr/1
  Mux3/1 -> H Filter Write Addr/1, testpoint/1
  Mux1/1 -> Bank 1 Read Addr/1
  Mux2/1 -> Bank 2 Read Addr/1
  1bit Cntr/1(q) -> Input Crossbar Switch/1
  Register7/1 -> 1bit Cntr/1(en)
  S-R FF/1(q) -> Inverter/1
  Start/1 -> S-R FF/1(s), [start]
  Register14/1 -> Counter/1
  Inverter/1 -> Register14/1
  [short_count] -> State/1(cnt)
  [start] -> State/2(start)
  State/3(we) -> L Filter WE/1, H Filter WE/1
  State/2(done) -> Done/1, [done]
  [done] -> S-R FF/2(r)
  short count/1 -> [short_count]
  testpoint/1 -> Signal To Workspace/1

== system DWT/Processor/Read Addr Crossbar ==
  note: Connect either A to A' and B to B'
      | or A to B' and B to A' based on
      | the signal "Cross".
  A : Inport
  B : Inport  Port=2
  Cross : Inport  Port=3
  Mux2 : xbsIndex_r4/Mux  inputs=2  en=off  latency=0  precision=Full  arith_type="Signed  (2's comp)"  n_bits=8  bin_pt=2  quantization=Truncate  overflow=Wrap  XmcBlockStatus=1  maskContainerNames=tabcontainer1  block_type=mux  block_config=sysgen:Mux_config
      settings: infoedit=[]
  Mux3 : xbsIndex_r4/Mux  inputs=2  en=off  latency=0  precision=Full  arith_type="Signed  (2's comp)"  n_bits=8  bin_pt=2  quantization=Truncate  overflow=Wrap  XmcBlockStatus=1  maskContainerNames=tabcontainer1  block_type=mux  block_config=sysgen:Mux_config
      settings: infoedit=[]
  A' : Outport  VectorParamsAs1DForOutWhenUnconnected=off
  B' : Outport  Port=2  VectorParamsAs1DForOutWhenUnconnected=off
  wires:
  Cross/1 -> Mux3/1, Mux2/1
  B/1 -> Mux2/3, Mux3/2
  A/1 -> Mux3/3, Mux2/2
  Mux3/1 -> B'/1
  Mux2/1 -> A'/1

== system DWT/Processor/WE Crossbar ==
  note: Connect either A to A' and B to B'
      | or A to B' and B to A' based on
      | the signal "Cross".
  A : Inport
  B : Inport  Port=2
  Cross : Inport  Port=3
  Mux2 : xbsIndex_r4/Mux  inputs=2  en=off  latency=1  precision=Full  arith_type="Signed  (2's comp)"  n_bits=8  bin_pt=2  quantization=Truncate  overflow=Wrap  XmcBlockStatus=1  maskContainerNames=tabcontainer1  block_type=mux  block_config=sysgen:Mux_config
      settings: infoedit=[]
  Mux3 : xbsIndex_r4/Mux  inputs=2  en=off  latency=1  precision=Full  arith_type="Signed  (2's comp)"  n_bits=8  bin_pt=2  quantization=Truncate  overflow=Wrap  XmcBlockStatus=1  maskContainerNames=tabcontainer1  block_type=mux  block_config=sysgen:Mux_config
      settings: infoedit=[]
  A' : Outport  VectorParamsAs1DForOutWhenUnconnected=off
  B' : Outport  Port=2  VectorParamsAs1DForOutWhenUnconnected=off
  wires:
  Mux2/1 -> A'/1
  Mux3/1 -> B'/1
  A/1 -> Mux2/2, Mux3/3
  B/1 -> Mux3/2, Mux2/3
  Cross/1 -> Mux2/1, Mux3/1

== system DWT/Processor/Write Addr Crossbar ==
  note: Connect either A to A' and B to B'
      | or A to B' and B to A' based on
      | the signal "Cross".
  A : Inport
  B : Inport  Port=2
  Cross : Inport  Port=3
  Mux2 : xbsIndex_r4/Mux  inputs=2  en=off  latency=1  precision=Full  arith_type="Signed  (2's comp)"  n_bits=8  bin_pt=2  quantization=Truncate  overflow=Wrap  XmcBlockStatus=1  maskContainerNames=tabcontainer1  block_type=mux  block_config=sysgen:Mux_config
      settings: infoedit=[]
  Mux3 : xbsIndex_r4/Mux  inputs=2  en=off  latency=1  precision=Full  arith_type="Signed  (2's comp)"  n_bits=8  bin_pt=2  quantization=Truncate  overflow=Wrap  XmcBlockStatus=1  maskContainerNames=tabcontainer1  block_type=mux  block_config=sysgen:Mux_config
      settings: infoedit=[]
  A' : Outport  VectorParamsAs1DForOutWhenUnconnected=off
  B' : Outport  Port=2  VectorParamsAs1DForOutWhenUnconnected=off
  wires:
  Mux2/1 -> A'/1
  Mux3/1 -> B'/1
  A/1 -> Mux2/2, Mux3/3
  B/1 -> Mux3/2, Mux2/3
  Cross/1 -> Mux2/1, Mux3/1

== system DWT/Processor/Memory Controller/1bit Cntr ==
  note: A 1-bit, synchronous counter.
      |
      | The Convert block does no work, it
      | just gives simulink a hint as to what
      | the feedback type is.
  en : Inport
  Convert : xbsIndex_r4/Convert  gui_display_data_type=Fixed-point  arith_type=Unsigned  n_bits=1  bin_pt=0  float_type=Single  exp_bits=8  fraction_bits=24  quantization=Truncate  overflow=Wrap  en=off  latency=0  pipeline=off  XmcBlockStatus=1  maskContainerNames=group2  block_type=convert  block_config=sysgen:Convert_config
  Inverter1 : xbsIndex_r4/Inverter  en=off  latency=0  XmcBlockStatus=1  maskContainerNames=group2  block_type=inv  block_config=sysgen:Inverter_config
  Register6 : xbsIndex_r4/Register  init=1  rst=off  en=on  XmcBlockStatus=1  maskContainerNames=tabcontainer1  block_type=register  block_config=sysgen:Register_config
  q : Outport  VectorParamsAs1DForOutWhenUnconnected=off
  wires:
  Inverter1/1 -> Register6/1
  Register6/1 -> Convert/1, q/1
  Convert/1 -> Inverter1/1
  en/1 -> Register6/2
